simulink model "SMD"  (R2018b)
settings: Solver=VariableStepAuto  StartTime=0.0  StopTime=10.0  RelTol=1e-3
values from neighbouring files (symbols this model uses):
  c = 1000    [baseVehicleData.mat]
  k = 10000    [baseVehicleData.mat]
  m = 250    [baseVehicleData.mat]
settings Model: Creator=Jamie  LastModifiedBy=Jamie

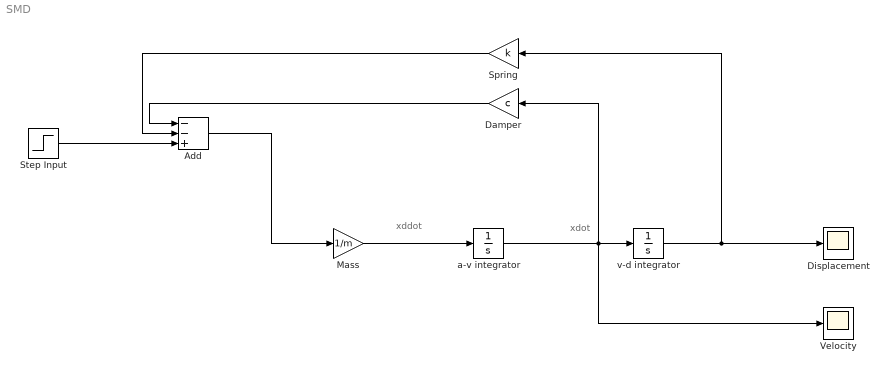
== system SMD ==
  note: xdot
  note: xddot
  "Add " : Sum  Inputs=--+
  Damper : Gain  Gain=c
  Displacement : Scope
  Mass : Gain  Gain=1/m
  Spring : Gain  Gain=k
  Step Input : Step  After=1000  SampleTime=0
  Velocity : Scope
  a-v integrator : Integrator  ContinuousStateAttributes=Velocity
  v-d integrator : Integrator  ContinuousStateAttributes=Position
  wires:
  Mass/1 -> a-v integrator/1
  a-v integrator/1 -> Velocity/1, Damper/1, v-d integrator/1
  v-d integrator/1 -> Displacement/1, Spring/1
  Spring/1 -> "Add "/2
  Damper/1 -> "Add "/1
  "Add "/1 -> Mass/1
  Step Input/1 -> "Add "/3
